simulink model "BPSK"  (Simulink 8.2)
settings: Solver=VariableStepDiscrete  StartTime=0.0  StopTime=50.0  RelTol=1e-3
libraries: commdigbbndpm3 x2, commsink2 x1
settings Model: Creator=yz10g11  LastModifiedBy=yz10g11
settings DebuggingCC: FcnCallInpInsideContextMsg=EnableAllAsWarning

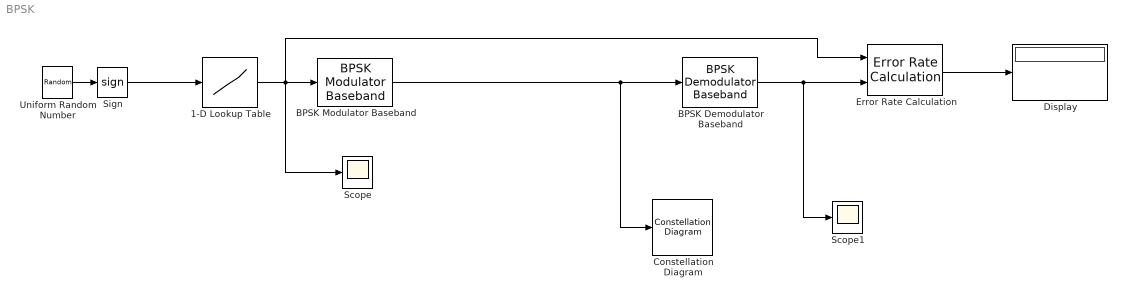
== system BPSK ==
  1-D Lookup Table : Lookup_n-D  NumberOfTableDimensions=1  BreakpointsForDimension1=[-1,0,1]  Table=[0,1,1]  RndMeth=Simplest  InputSameDT=on
  BPSK Demodulator Baseband : commdigbbndpm3/BPSK Demodulator Baseband  Ph=0  DecType=Hard decision  VarSource=Dialog  Variance=1  outDtype=Inherit via internal rule  derotateFactorWordLen=16
  BPSK Modulator Baseband : commdigbbndpm3/BPSK Modulator Baseband  Ph=0  outDtype=double  outWordLen=16  outUDDataType=sfix(16)  outFracLenMode=Best precision  outFracLen=15
  Constellation Diagram : ConstellationDiagram  ScopeSpecification=DataTag0
      settings: CopyFcn=scopeextensions.ScopeBlock.onCoreBlockCopy(gcbh);  DeleteFcn=scopeextensions.ScopeBlock.callback(gcbh, 'onBlockDelete');  PreSaveFcn=scopeextensions.ScopeBlock.callback(gcbh, 'onModelSave');  NameChangeFcn=scopeextensions.ScopeBlock.callback(gcbh, 'onBlockRename');  DestroyFcn=scopeextensions.ScopeBlock.onBlockDestroy(gcbh)  CloseFcn=scopeextensions.ScopeBlock.callback(gcbh, 'onBlockClose');  PreDeleteFcn=scopeextensions.ScopeBlock.callback(gcbh, 'onBlockPreDelete');
  Display : Display
  Error Rate Calculation : commsink2/Error Rate Calculation  N=0  st_delay=0  cp_mode=Entire frame  subframe=[]  PMode=Port  WsName=ErrorVec  RsMode2=off  stop=off  numErr=100  maxBits=1e6
  Scope : Scope
  Scope1 : Scope
  Sign : Signum
  Uniform Random Number : UniformRandomNumber  SampleTime=1
  wires:
  Uniform Random Number/1 -> Sign/1
  Sign/1 -> 1-D Lookup Table/1
  1-D Lookup Table/1 -> Error Rate Calculation/1, Scope/1, BPSK Modulator Baseband/1
  BPSK Demodulator Baseband/1 -> Scope1/1, Error Rate Calculation/2
  Error Rate Calculation/1 -> Display/1
  BPSK Modulator Baseband/1 -> Constellation Diagram/1, BPSK Demodulator Baseband/1
